simulink model "Team6_1"  (R2018b)
settings: Solver=VariableStepAuto  StartTime=0.0  StopTime=10  RelTol=1e-3
undefined symbols (not defined in the file): sigbuilder_block
(part 1 of 2)
settings Model: EnablePacing=on  PacingRate=0.500000  Creator=99003175  LastModifiedBy=Hp
settings DataIOCC: ReturnWorkspaceOutputs=on
settings OptimizationCC: DefaultUnderspecifiedDataType=single
settings DebuggingCC: SignalInfNanChecking=warning  UniqueDataStoreMsg=error  AssertControl=DisableAll  StrictBusMsg=ErrorOnBusTreatedAsVector  SFUndirectedBroadcastEventsDiag=error
settings SFSimCC: CompileTimeRecursionLimit=0  EnableRuntimeRecursion=off  MATLABDynamicMemAlloc=off

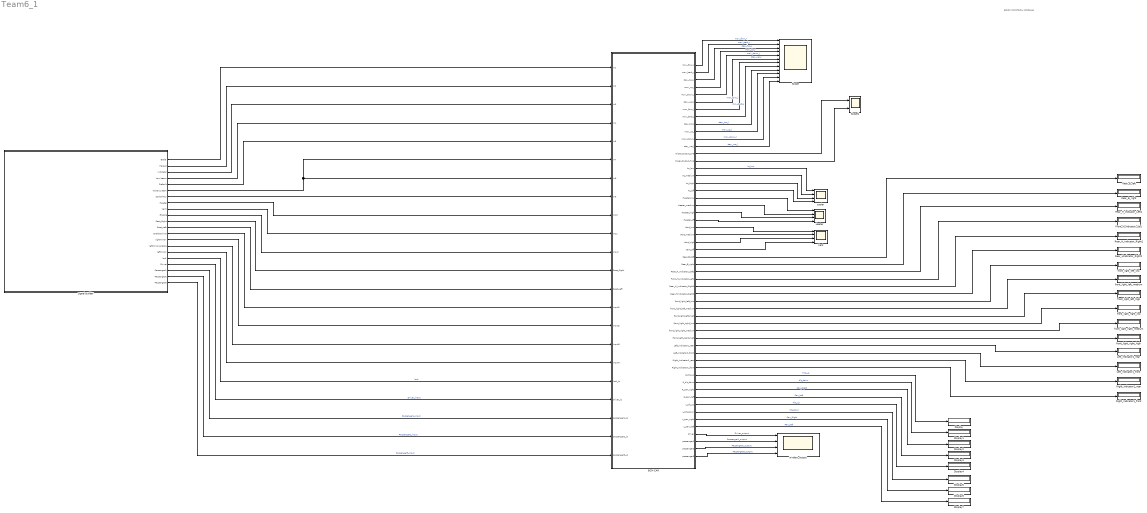
== system Team6_1 ==
  note: BODY CONTROL MODULE
  BCM CAR : Subsystem
  Display{,1..7} (8 alike) : Display
  Front_H_Indicator_Lef1 : Display
  Heater : Scope  NumInputPorts=4
  Left_Indicator1_front : Display
  Left_Indicator1_rear : Display
  Rear_B_left : Display
  Rear_B_right : Display
  Rear_HIndicator_Right2 : Display
  Rear_H_Indicator_Left1 : Display
  Rear_H_Indicator_Right1 : Display
  Right_Indicator1_front : Display
  Right_Indicator1_rear : Display
  Scope : Scope  NumInputPorts=12
  Scope1 : Scope  NumInputPorts=2
  Signal Builder : Subsystem  Tag=STV Subsys  LoadFcn=sigbuilder_block('load');  StartFcn=sigbuilder_block('start');  StopFcn=sigbuilder_block('stop');  ClipboardFcn=sigbuilder_block('clipboard');  mask(Sigbuilder block){tuvar=[0:10]}
      mask help: Simulink:masks:SigbuilderBlock_MD
      mask init:
      | if ~strcmp(get_param(bdroot(gcbh),'SimulationStatus'),'stopped') tuvar = sigbuilder_block('maskInit'); end
      settings: CopyFcn=sigbuilder_block('copy');  DeleteFcn=sigbuilder_block('delete');  ModelCloseFcn=sigbuilder_block('modelClose');  PreSaveFcn=sigbuilder_block('preSave');  PauseFcn=sigbuilder_block('pause');  ContinueFcn=sigbuilder_block('continue');  NameChangeFcn=sigbuilder_block('namechange');  OpenFcn=sigbuilder_block('open',[6 46.5 1188 465.75 ]);  CloseFcn=sigbuilder_block('close');
      mask Display: plot(0, 0, 100, 100,[2, 2, 32, 32, 2], [68, 8, 8, 68, 68],[32, 2], [38, 38], [32, 19, 2],[53, 60, 44], [32, 17, 17, 2],[16, 16, 31, 31]);txt = getActiveGroup(gcbh);text(2, 100, txt,'verticalAlignment', 'top');
  Vent : Scope  NumInputPorts=4
  cooler : Scope  NumInputPorts=4
  front_light_left_high : Display
  front_light_left_low : Display
  front_light_left_medium : Display
  front_light_right_high : Display
  front_light_right_low : Display
  front_light_right_medium : Display
  window_output : Scope  NumInputPorts=4
  wires:
  Signal Builder/9(Vent) -> BCM CAR/10(In11)
  Signal Builder/16(leftmirror) -> BCM CAR/17(Input4)
  BCM CAR/46(R_pan_left) -> Display3/1  "Pan_left"
  Signal Builder/15(leftmirror enable) -> BCM CAR/16(Input3)
  Signal Builder/14(rightmirror) -> BCM CAR/15(Input2)
  BCM CAR/43(R_tilt_up) -> Display/1  "Tilt_up"
  BCM CAR/45(R_pan_right) -> Display2/1  "Pan_Right"
  Signal Builder/13(enablemirror) -> BCM CAR/14(Input1)
  BCM CAR/44(R_tilt_down) -> Display1/1  "tilt_down"
  Signal Builder/6(Wiper system) -> BCM CAR/6(In7), BCM CAR/7(In8)
  Signal Builder/5(Default) -> BCM CAR/5(In5)
  Signal Builder/12(Seat_Left) -> BCM CAR/13(Seat_Left)
  Signal Builder/4(Low beam) -> BCM CAR/4(In4)
  Signal Builder/1(Brake) -> BCM CAR/1(In1)
  Signal Builder/7(Cooler(AC)) -> BCM CAR/8(In9)
  Signal Builder/3(Indicator) -> BCM CAR/3(In3)
  Signal Builder/10(Enable) -> BCM CAR/11(Input)
  Signal Builder/11(Seat_Right) -> BCM CAR/12(Seat_Right)
  Signal Builder/2(Hazard) -> BCM CAR/2(In2)
  Signal Builder/8(Heater) -> BCM CAR/9(In10)
  BCM CAR/27(Rear_B_left) -> Rear_B_left/1
  BCM CAR/26(Vent_off) -> Vent/4
  BCM CAR/32(Rear_HIndicator_Right2) -> Rear_HIndicator_Right2/1
  BCM CAR/9(stay_hor_l) -> Scope/9  "stay_hor_l"
  BCM CAR/33(front_light_left_low) -> front_light_left_low/1
  BCM CAR/39(Left_Indicator1_rear) -> Left_Indicator1_rear/1
  BCM CAR/30(Front_H_Indicator_Lef1) -> Front_H_Indicator_Lef1/1
  BCM CAR/17(Ac_high) -> cooler/3
  BCM CAR/36(front_light_right_low) -> front_light_right_low/1
  BCM CAR/42(Right_Indicator1_front) -> Right_Indicator1_front/1
  BCM CAR/35(front_light_left_high) -> front_light_left_high/1
  BCM CAR/38(front_light_right_high) -> front_light_right_high/1
  BCM CAR/28(Rear_B_right) -> Rear_B_right/1
  BCM CAR/13(Wiper_Output_one) -> Scope1/1
  BCM CAR/29(Rear_H_Indicator_Left1) -> Rear_H_Indicator_Left1/1
  BCM CAR/31(Rear_H_Indicator_Right1) -> Rear_H_Indicator_Right1/1
  BCM CAR/2(mov_back_r) -> Scope/2  "mov_back_r"
  BCM CAR/3(stay_hor_r) -> Scope/3  "stay_hor_r"
  BCM CAR/37(front_light_right_medium) -> front_light_right_medium/1
  BCM CAR/8(mov_back_l) -> Scope/8  "mov_back_l"
  BCM CAR/34(front_light_left_medium) -> front_light_left_medium/1
  BCM CAR/14(Wiper_Output_Two) -> Scope1/2
  BCM CAR/18(Ac_off) -> cooler/4
  BCM CAR/41(Right_Indicator1_rear) -> Right_Indicator1_rear/1
  BCM CAR/40(Left_Indicator1_front) -> Left_Indicator1_front/1
  BCM CAR/25(Vent_high) -> Vent/3
  BCM CAR/24(Vent_medium) -> Vent/2
  BCM CAR/15(Ac_low) -> cooler/1  "Ac_low"
  BCM CAR/23(Vent_low) -> Vent/1
  BCM CAR/1(mov_forw_r) -> Scope/1  "mov_forw_r"
  BCM CAR/22(Heater_off) -> Heater/4
  BCM CAR/12(stay_ver_l) -> Scope/12  "stay_ver_l"
  BCM CAR/21(Heater_high) -> Heater/3
  BCM CAR/11(mov_down_l) -> Scope/11  "mov_down_l"
  BCM CAR/20(Heater_medium) -> Heater/2
  BCM CAR/19(Heater_low) -> Heater/1
  BCM CAR/16(Ac_medium) -> cooler/2
  BCM CAR/5(mov_down_r) -> Scope/5  "mov_down_r"
  BCM CAR/4(mov_up_r) -> Scope/4  "mov_up_r"
  BCM CAR/6(stay_ver_r) -> Scope/6  "stay_ver_r"
  BCM CAR/7(mov_forw_l) -> Scope/7  "mov_forw_l"
  BCM CAR/10(mov_up_l) -> Scope/10  "mov_up_l"
  BCM CAR/47(L_tilt_up) -> Display4/1  "Tilt_up"
  BCM CAR/50(L_pan_left) -> Display7/1  "Pan_left"
  BCM CAR/49(L_pan_right) -> Display6/1  "Pan_Right"
  BCM CAR/48(L_tilt_down) -> Display5/1  "tilt_down"
  Signal Builder/17(lock) -> BCM CAR/18(lock_ip)  "lock"
  Signal Builder/18(Driver) -> BCM CAR/19(driver_ip)  "Driver_input"
  Signal Builder/19(Passenger1) -> BCM CAR/20(passenger1_ip)  "Passenger1_input"
  Signal Builder/20(Passenger2) -> BCM CAR/21(passenger2_ip)  "Passenger2_input"
  Signal Builder/21(Passenger3) -> BCM CAR/22(passenger3_ip)  "Passenger3_input"
  BCM CAR/51(driver) -> window_output/1  "Driver_output"
  BCM CAR/52(passenger1) -> window_output/2  "Passenger1_output"
  BCM CAR/53(passenger2) -> window_output/3  "Passenger2_output"
  BCM CAR/54(passenger3) -> window_output/4  "Passenger3_output"

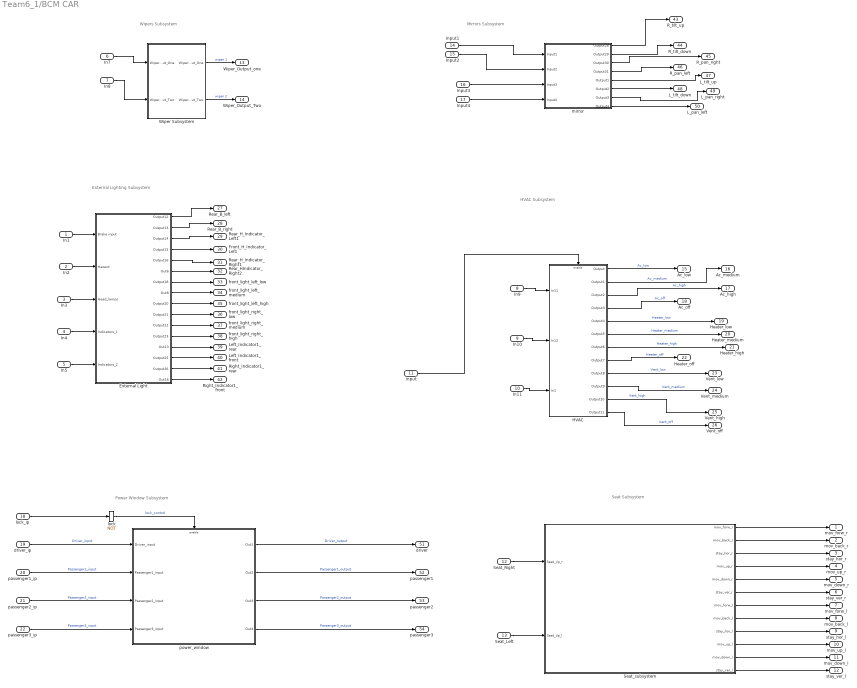
== system Team6_1/BCM CAR ==
  note: Seat Subsystem
  note: External Lighting Subsystem
  note: HVAC Subsystem
  note: Mirrors Subsystem
  note: Wipers Subsystem
  note: Power Window Subsystem
  In1 : Inport
  In2 : Inport  Port=2
  In3 : Inport  Port=3
  In4 : Inport  Port=4
  In5 : Inport  Port=5
  In7 : Inport  Port=6
  In8 : Inport  Port=7
  In9 : Inport  Port=8
  In10 : Inport  Port=9
  In11 : Inport  Port=10
  Input : Inport  Port=11
  Seat_Right : Inport  Port=12
  Seat_Left : Inport  Port=13
  Input1 : Inport  Port=14
  Input2 : Inport  Port=15
  Input3 : Inport  Port=16
  Input4 : Inport  Port=17
  lock_ip : Inport  Port=18
  driver_ip : Inport  Port=19
  passenger1_ip : Inport  Port=20
  passenger2_ip : Inport  Port=21
  passenger3_ip : Inport  Port=22
  External Light : Subsystem  TreatAsAtomicUnit=on
  HVAC : Subsystem
  Seat_subsystem : Subsystem  TreatAsAtomicUnit=on
  Wiper Subsystem : Subsystem  TreatAsAtomicUnit=on
  lock : Logic  Operator=NOT  IconShape=distinctive  AllPortsSameDT=off  OutDataTypeStr=boolean
  mirror : Subsystem  TreatAsAtomicUnit=on
  power_window : Subsystem
  mov_forw_r : Outport
  mov_back_r : Outport  Port=2
  stay_hor_r : Outport  Port=3
  mov_up_r : Outport  Port=4
  mov_down_r : Outport  Port=5
  stay_ver_r : Outport  Port=6
  mov_forw_l : Outport  Port=7
  mov_back_l : Outport  Port=8
  stay_hor_l : Outport  Port=9
  mov_up_l : Outport  Port=10
  mov_down_l : Outport  Port=11
  stay_ver_l : Outport  Port=12
  Wiper_Output_one : Outport  Port=13
  Wiper_Output_Two : Outport  Port=14
  Ac_low : Outport  Port=15
  Ac_medium : Outport  Port=16
  Ac_high : Outport  Port=17
  Ac_off : Outport  Port=18
  Heater_low : Outport  Port=19
  Heater_medium : Outport  Port=20
  Heater_high : Outport  Port=21
  Heater_off : Outport  Port=22
  Vent_low : Outport  Port=23
  Vent_medium : Outport  Port=24
  Vent_high : Outport  Port=25
  Vent_off : Outport  Port=26
  Rear_B_left : Outport  Port=27
  Rear_B_right : Outport  Port=28
  Rear_H_Indicator_Left1 : Outport  Port=29
  Front_H_Indicator_Lef1 : Outport  Port=30
  Rear_H_Indicator_Right1 : Outport  Port=31
  Rear_HIndicator_Right2 : Outport  Port=32
  front_light_left_low : Outport  Port=33
  front_light_left_medium : Outport  Port=34
  front_light_left_high : Outport  Port=35
  front_light_right_low : Outport  Port=36
  front_light_right_medium : Outport  Port=37
  front_light_right_high : Outport  Port=38
  Left_Indicator1_rear : Outport  Port=39
  Left_Indicator1_front : Outport  Port=40
  Right_Indicator1_rear : Outport  Port=41
  Right_Indicator1_front : Outport  Port=42
  R_tilt_up : Outport  Port=43
  R_tilt_down : Outport  Port=44
  R_pan_right : Outport  Port=45
  R_pan_left : Outport  Port=46
  L_tilt_up : Outport  Port=47
  L_tilt_down : Outport  Port=48
  L_pan_right : Outport  Port=49
  L_pan_left : Outport  Port=50
  driver : Outport  Port=51
  passenger1 : Outport  Port=52
  passenger2 : Outport  Port=53
  passenger3 : Outport  Port=54
  wires:
  In7/1 -> Wiper Subsystem/1(Wiper_Input_One)
  HVAC/6(Output5) -> Heater_medium/1  "Heater_medium"
  HVAC/3(Output2) -> Ac_high/1  "Ac_high"
  In1/1 -> External Light/1(Brake input)
  HVAC/7(Output6) -> Heater_high/1  "Heater_high"
  In4/1 -> External Light/4(Indicators_1)
  HVAC/4(Output3) -> Ac_off/1  "Ac_off"
  In8/1 -> Wiper Subsystem/2(Wiper_Input_Two)
  In9/1 -> HVAC/1(In11)
  HVAC/2(Output1) -> Ac_medium/1  "Ac_medium"
  HVAC/5(Output4) -> Heater_low/1  "Heater_low"
  In10/1 -> HVAC/2(In12)
  HVAC/12(Output11) -> Vent_off/1  "Vent_off"
  HVAC/10(Output9) -> Vent_medium/1  "Vent_medium"
  In5/1 -> External Light/5(Indicators_2)
  HVAC/8(Output7) -> Heater_off/1  "Heater_off"
  HVAC/11(Output10) -> Vent_high/1  "Vent_high"
  HVAC/1(Output) -> Ac_low/1  "Ac_low"
  HVAC/9(Output8) -> Vent_low/1  "Vent_low"
  In11/1 -> HVAC/3(In1)
  In3/1 -> External Light/3(Head_lamps)
  In2/1 -> External Light/2(Hazard)
  Input/1 -> HVAC/Enable
  Seat_subsystem/7(mov_forw_l) -> mov_forw_l/1
  Seat_subsystem/8(mov_back_l) -> mov_back_l/1
  Seat_subsystem/6(stay_ver_r) -> stay_ver_r/1
  Seat_Right/1 -> Seat_subsystem/1(Seat_i/p_r)
  Seat_Left/1 -> Seat_subsystem/2(Seat_i/p_l)
  Seat_subsystem/9(stay_hor_l) -> stay_hor_l/1
  Seat_subsystem/11(mov_down_l) -> mov_down_l/1
  Seat_subsystem/12(stay_ver_l) -> stay_ver_l/1
  Seat_subsystem/4(mov_up_r) -> mov_up_r/1
  Seat_subsystem/1(mov_forw_r) -> mov_forw_r/1
  Seat_subsystem/5(mov_down_r) -> mov_down_r/1
  Seat_subsystem/3(stay_hor_r) -> stay_hor_r/1
  Seat_subsystem/10(mov_up_l) -> mov_up_l/1
  Seat_subsystem/2(mov_back_r) -> mov_back_r/1
  Wiper Subsystem/1(Wiper_Output_One) -> Wiper_Output_one/1  "wiper 1"
  Wiper Subsystem/2(Wiper_Output_Two) -> Wiper_Output_Two/1  "wiper 2"
  External Light/1(Output12) -> Rear_B_left/1
  External Light/2(Output13) -> Rear_B_right/1
  External Light/3(Output14) -> Rear_H_Indicator_Left1/1
  External Light/4(Output15) -> Front_H_Indicator_Lef1/1
  External Light/5(Output16) -> Rear_H_Indicator_Right1/1
  External Light/6(Out6) -> Rear_HIndicator_Right2/1
  External Light/7(Output18) -> front_light_left_low/1
  External Light/8(Out8) -> front_light_left_medium/1
  External Light/9(Output20) -> front_light_left_high/1
  External Light/10(Output21) -> front_light_right_low/1
  External Light/11(Output22) -> front_light_right_medium/1
  External Light/12(Output23) -> front_light_right_high/1
  External Light/13(Out13) -> Left_Indicator1_rear/1
  External Light/14(Output25) -> Left_Indicator1_front/1
  External Light/15(Output26) -> Right_Indicator1_rear/1
  External Light/16(Out16) -> Right_Indicator1_front/1
  Input1/1 -> mirror/1(Input1)
  Input2/1 -> mirror/2(Input2)
  mirror/1(Output28) -> R_tilt_up/1
  mirror/3(Output30) -> R_pan_right/1
  mirror/2(Output29) -> R_tilt_down/1
  mirror/4(Output31) -> R_pan_left/1
  mirror/5(Output1) -> L_tilt_up/1
  mirror/6(Output2) -> L_tilt_down/1
  mirror/7(Output3) -> L_pan_right/1
  mirror/8(Output4) -> L_pan_left/1
  Input4/1 -> mirror/4(Input4)
  Input3/1 -> mirror/3(Input3)
  lock/1 -> power_window/Enable  "lock_control"
  passenger1_ip/1 -> power_window/2(Passenger1_input)  "Passenger1_input"
  power_window/3(Out3) -> passenger2/1  "Passenger2_output"
  power_window/2(Out2) -> passenger1/1  "Passenger1_output"
  passenger3_ip/1 -> power_window/4(Passenger3_input)  "Passenger3_input"
  passenger2_ip/1 -> power_window/3(Passenger2_input)  "Passenger2_input"
  driver_ip/1 -> power_window/1(Driver_input)  "Driver_input"
  power_window/1(Out1) -> driver/1  "Driver_output"
  power_window/4(Out4) -> passenger3/1  "Passenger3_output"
  lock_ip/1 -> lock/1

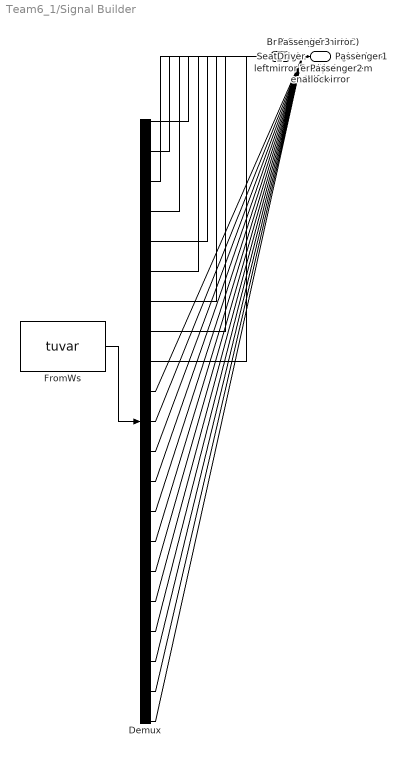
== system Team6_1/Signal Builder ==
  Demux : Demux  Tag=STV Demux  Outputs=21
      settings: DisplayOption=none
  FromWs : FromWorkspace  Tag=STV FromWs  VariableName=tuvar
      SigBuilderData=|
      | common.afterFinalStr = 'Extrapolate'
      | common.sampleTime = 0
      | dataSet.timeRange = [0 10]
      | dataSet.name = 'Group 1'
      | sbobj.Groups.Name = 'Group 1'
      | sbobj.Groups.Signals(1).Name = 'Brake'
      | sbobj.Groups.Signals(1).XData = [0 3 3 6 6 10]
      | sbobj.Groups.Signals(1).YData = [0 0 1 1 0 0]
      | sbobj.Groups.Signals(2).Name = 'Hazard'
      | sbobj.Groups.Signals(2).XData = [0 0.5 0.5 1 1 1.5 1.5 2 2 2.5 2.5 3 3 3.5 3.5 4 4 4.5 4.5 5 5 5.5 5.5 6 6 6.5 6.5 7 7 7.5 7.5 8 8 8.5 8.5 9 9 9.5 9.5 10]
      | sbobj.Groups.Signals(2).YData = [2 2 0 0 2 2 0 0 2 2 0 0 2 2 0 0 2 2 0 0 2 2 0 0 2 2 0 0 2 2 0 0 2 2 0 0 2 2 0 0]
      | sbobj.Groups.Signals(3).Name = 'Indicator'
      | sbobj.Groups.Signals(3).XData = [0 1 1 4.02 4.02 10]
      | sbobj.Groups.Signals(3).YData = [0 0 1.05 1.05 0 0]
      | sbobj.Groups.Signals(4).Name = 'Low beam'
      | sbobj.Groups.Signals(4).XData = [0 5.96 5.96 7.96 7.96 10]
      | sbobj.Groups.Signals(4).YData = [0 0 1.05 1.05 0 0]
      | sbobj.Groups.Signals(5).Name = 'Default'
      | sbobj.Groups.Signals(5).XData = [0 1 1 8 8 10]
      | sbobj.Groups.Signals(5).YData = [0 0 -0.4 -0.4 1 1]
      | sbobj.Groups.Signals(6).Name = 'Wiper system'
      | sbobj.Groups.Signals(6).XData = [0 0.5 1 1 1.5 1.5 2 2 2.5 2.5 3 3 3.5 3.5 4 4 4.5 4.5 5 5 5.5 5.5 6 6 6.5 6.5 7 7 7.5 7.5 8 8 8.5 8.5 9 9 9.5 9.5 10]
      | sbobj.Groups.Signals(6).YData = [3 3 3 2.5 1 2 2 0.85 0.85 1.95 1.95 1 1 1.1 1.1 2 2 0.95 0.95 0.8 0.8 0.95 0.95 2 2 0.8 0.8 2.5 2.5 2.05 2.05 0.95 0.95 0.6 0.6 0 0 5 5]
      | sbobj.Groups.Signals(7).Name = 'Cooler(AC)'
      | sbobj.Groups.Signals(7).XData = [0 0.5 0.5 1 1 1.5 1.5 2 2 2.5 2.5 3 3 3.5 3.5 4 4 4.5 4.5 5 5 5.5 5.5 6 6 6.5 6.5 7 7 7.5 7.5 8 8 8.5 8.5 9 9 9.5 10]
      | sbobj.Groups.Signals(7).YData = [2 2 1 1 0 0 0.9 0.9 2 2 3 3 1.2 1.2 2.2 2.2 0.9 0.9 0 0 2 2 3 3 2 2 0 0 2 2 0 0 2 2 0 0 2 2 2]
      | sbobj.Groups.Signals(8).Name = 'Heater'
      | sbobj.Groups.Signals(8).XData = [0 0.5 0.5 1 1 1.5 1.5 2 2 2.5 2.5 3 3 3.5 3.5 4 4 4.5 4.5 5 5 5.5 5.5 6 6 6.5 6.5 7 7 7.5 7.5 8 8 8.5 8.5 9 9 9.5 9.5 10]
      | sbobj.Groups.Signals(8).YData = [2 2 0.9 0.9 0 0 0.8 0.8 2 2 0 0 3 3 1 1 2 2 0 0 1 1 0 0 3 3 2 2 3 3 0 0 2 2 0 0 2 2 1 1]
      | sbobj.Groups.Signals(9).Name = 'Vent'
      | sbobj.Groups.Signals(9).XData = [0 0.5 0.5 1 1 1.5 1.5 2 2 2.5 2.5 3 3 3.5 3.5 4 4 4.5 4.5 5 5 5.5 5.5 6 6 6.5 6.5 7 7 7.5 7.5 8 8 8.5 8.5 9 9 9.5 9.5 10]
      | sbobj.Groups.Signals(9).YData = [2 2 1.1 1.1 0 0 1.8 1.8 0.9 0.9 1.9 1.9 0.1 0.1 1.8 1.8 -0.2 -0.2 1.4 1.4 3 3 0 0 2 2 3 3 2 2 1 1 2 2 0 0 3 3 1.1 1.1]
      | sbobj.Groups.Signals(10).Name = 'Enable'
      | sbobj.Groups.Signals(10).XData = [0 10]
      | sbobj.Groups.Signals(10).YData = [1 1]
      | sbobj.Groups.Signals(11).Name = 'Seat_Right'
      | sbobj.Groups.Signals(11).XData = [0 0.5 0.5 1 1 1.5 1.5 2 2 2.5 2.5 3 3 3.5 3.5 4 4 4.5 4.5 5 5 5.5 5.5 6 6 6.5 6.5 7 7 7.5 7.5 8 8 8.5 8.5 9 9 9.5 9.5 10]
      | sbobj.Groups.Signals(11).YData = [1 1 0 0 1 1 -1 -1 1 1 0 0 1 1 0 0 1 1 0 0 2 2 0 0 2 2 0 0 2 2 0 0 2 2 0 0 2 2 0 0]
      | sbobj.Groups.Signals(12).Name = 'Seat_Left'
      | sbobj.Groups.Signals(12).XData = [0 0.5 0.5 1 1 1.5 1.5 2 2 2.5 2.5 3 3 3.5 3.5 4 4 4.5 4.5 5 5 5.5 5.5 6 6 6.5 6.5 7 7 7.5 7.5 8 8 8.5 8.5 9 9 9.5 9.5 10]
      | sbobj.Groups.Signals(12).YData = [1 1 0 0 -1 -1 0 0 1 1 0 0 -1 -1 0 0 1 1 0 0 2 2 0 0 2 2 0 0 2 2 0 0 2 2 0 0 2 2 0 0]
      | sbobj.Groups.Signals(13).Name = 'enablemirror'
      | sbobj.Groups.Signals(13).XData = [0 0.5 0.5 1 1 1.5 1.5 2 2.5 3 3 3.5 3.5 4 4 4.5 4.5 5 5 5.5 5.5 6 6 6.5 6.5 7 7 7.5 7.5 8 8 8.5 8.5 9 9 9.5 9.5 10]
      | sbobj.Groups.Signals(13).YData = [1 1 0 0 -1 -1 0 0 0 0 1 1 0 0 -1 -1 0 0 2 2 0 0 2 2 0 0 2 2 0 0 2 2 0 0 2 2 0 0]
      | sbobj.Groups.Signals(14).Name = 'rightmirror'
      | sbobj.Groups.Signals(14).XData = [0 0.5 0.5 1 1 1.5 1.5 2 2 2.5 2.5 3 3 3.5 3.5 4 4 4.5 4.5 5 5 5.5 5.5 6 6 6.5 6.5 7 7 7.5 7.5 8 8 8.5 8.5 9 9 9.5 9.5 10]
      | sbobj.Groups.Signals(14).YData = [2 2 0 0 -1 -1 1 1 2 2 0 0 1 1 -1 -1 2 2 0 0 1 1 -1 -1 2 2 1 1 2 2 0 0 1 1 0 0 -1 -1 1 1]
      | sbobj.Groups.Signals(15).Name = 'leftmirror enable'
      | sbobj.Groups.Signals(15).XData = [0 10]
      | sbobj.Groups.Signals(15).YData = [1 1]
      | sbobj.Groups.Signals(16).Name = 'leftmirror'
      | sbobj.Groups.Signals(16).XData = [0 0.5 0.5 1 1 1.5 1.5 2 2 2.5 2.5 3 3 3.5 3.5 4 4 4.5 4.5 5 5 5.5 5.5 6 6 6.5 6.5 7 7 7.5 7.5 8 8 8.5 8.5 9 9 9.5 9.5 10]
      | sbobj.Groups.Signals(16).YData = [2 2 0 0 2 2 0 0 2 2 0 0 2 2 0 0 2 2 0 0 2 2 0 0 2 2 0 0 2 2 0 0 2 2 0 0 2 2 0 0]
      | sbobj.Groups.Signals(17).Name = 'lock'
      | sbobj.Groups.Signals(17).XData = [0 0.5 1 1 1.5 1.5 2 2 2.5 2.5 3 3 3.5 3.5 4 4 4.5 4.5 5 5 5.5 5.5 6 6 6.5 6.5 7 7 7.5 7.5 8 8 8.5 8.5 9 9 9.5 9.5 10]
      | sbobj.Groups.Signals(17).YData = [0 0 0 1 1 0 0 1 1 0 0 2 2 0 0 2 2 0 0 2 2 0 0 2 2 0 0 2 2 0 0 2 2 0 0 2 2 0 0]
      | sbobj.Groups.Signals(18).Name = 'Driver'
      | sbobj.Groups.Signals(18).XData = [0 0.5 1 1 1.5 1.5 2 2 2.5 2.5 3 3 3.5 3.5 4 4 4.5 4.5 5 5 5.5 5.5 6 6 6.5 6.5 7 7 7.5 7.5 8 8 8.5 8.5 9 9 9.5 9.5 10]
      | sbobj.Groups.Signals(18).YData = [1 1 1 2 2 0 0 3 3 0 0 4 4 0 0 2 2 0 0 2 2 0 0 2 2 0 0 2 2 0 0 2 2 0 0 2 2 0 0]
      | sbobj.Groups.Signals(19).Name = 'Passenger1'
      | sbobj.Groups.Signals(19).XData = [0 0.5 0.5 1 1 1.5 1.5 2 2 2.5 2.5 3 3 3.5 3.5 4 4 4.5 4.5 5 5 5.5 5.5 6 6 6.5 6.5 7 7 7.5 7.5 8 8 8.5 8.5 9 9 9.5 9.5 10]
      | sbobj.Groups.Signals(19).YData = [1 1 0 0 2 2 0 0 3 3 0 0 4 4 0 0 2 2 0 0 2 2 0 0 2 2 0 0 2 2 0 0 2 2 0 0 2 2 0 0]
      | sbobj.Groups.Signals(20).Name = 'Passenger2'
      | sbobj.Groups.Signals(20).XData = [0 0.5 0.5 1 1 1.5 1.5 2 2 2.5 2.5 3 3 3.5 3.5 4 4 4.5 4.5 5 5 5.5 5.5 6 6 6.5 6.5 7 7 7.5 7.5 8 8 8.5 8.5 9 9 9.5 9.5 10]
      | sbobj.Groups.Signals(20).YData = [1 1 0 0 2 2 0 0 3 3 0 0 4 4 0 0 2 2 0 0 2 2 0 0 2 2 0 0 2 2 0 0 2 2 0 0 2 2 0 0]
      | sbobj.Groups.Signals(21).Name = 'Passenger3'
      | sbobj.Groups.Signals(21).XData = [0 0.5 0.5 1 1 1.5 1.5 2 2 2.5 2.5 3 3 3.5 3.5 4 4 4.5 4.5 5 5 5.5 5.5 6 6 6.5 6.5 7 7 7.5 7.5 8 8 8.5 8.5 9 9 9.5 9.5 10]
      | sbobj.Groups.Signals(21).YData = [1 1 0 0 2 2 0 0 3 3 0 0 4 4 0 0 2 2 0 0 2 2 0 0 2 2 0 0 2 2 0 0 2 2 0 0 2 2 0 0]
  Brake : Outport  Tag=STV Outport
  Hazard : Outport  Tag=STV Outport  Port=2
  Indicator : Outport  Tag=STV Outport  Port=3
  Low beam : Outport  Tag=STV Outport  Port=4
  Default : Outport  Tag=STV Outport  Port=5
  Wiper system : Outport  Tag=STV Outport  Port=6
  Cooler(AC) : Outport  Tag=STV Outport  Port=7
  Heater : Outport  Tag=STV Outport  Port=8
  Vent : Outport  Tag=STV Outport  Port=9
  Enable : Outport  Tag=STV Outport  Port=10
  Seat_Right : Outport  Tag=STV Outport  Port=11
  Seat_Left : Outport  Tag=STV Outport  Port=12
  enablemirror : Outport  Tag=STV Outport  Port=13
  rightmirror : Outport  Tag=STV Outport  Port=14
  leftmirror enable : Outport  Tag=STV Outport  Port=15
  leftmirror : Outport  Tag=STV Outport  Port=16
  lock : Outport  Tag=STV Outport  Port=17
  Driver : Outport  Tag=STV Outport  Port=18
  Passenger1 : Outport  Tag=STV Outport  Port=19
  Passenger2 : Outport  Tag=STV Outport  Port=20
  Passenger3 : Outport  Tag=STV Outport  Port=21
  wires:
  Demux/1 -> Brake/1
  FromWs/1 -> Demux/1
  Demux/2 -> Hazard/1
  Demux/3 -> Indicator/1
  Demux/4 -> Low beam/1
  Demux/5 -> Default/1
  Demux/6 -> Wiper system/1
  Demux/7 -> Cooler(AC)/1
  Demux/8 -> Heater/1
  Demux/9 -> Vent/1
  Demux/10 -> Enable/1
  Demux/11 -> Seat_Right/1
  Demux/12 -> Seat_Left/1
  Demux/13 -> enablemirror/1
  Demux/14 -> rightmirror/1
  Demux/15 -> leftmirror enable/1
  Demux/16 -> leftmirror/1
  Demux/17 -> lock/1
  Demux/18 -> Driver/1
  Demux/19 -> Passenger1/1
  Demux/20 -> Passenger2/1
  Demux/21 -> Passenger3/1

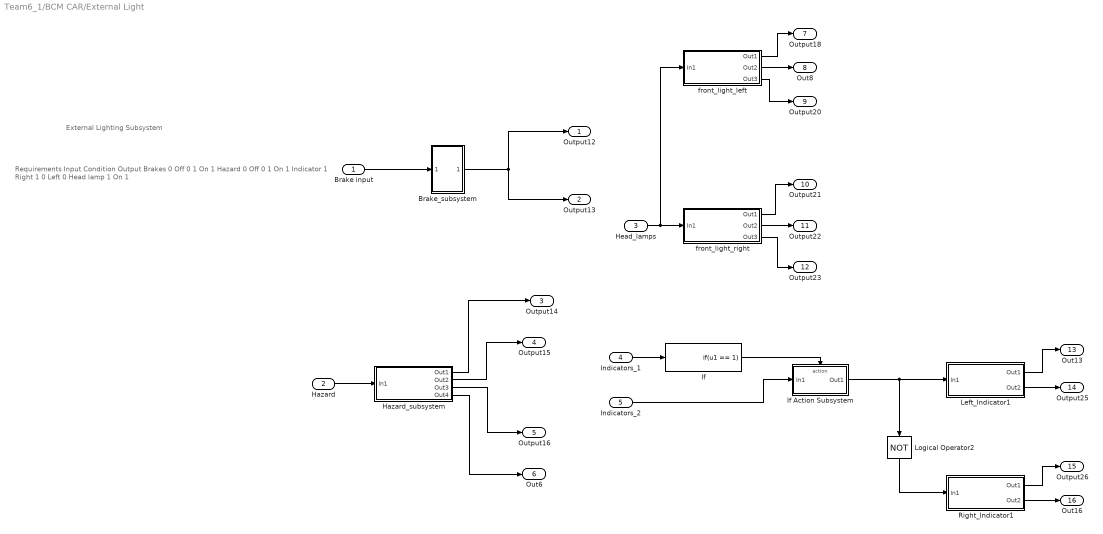
== system Team6_1/BCM CAR/External Light ==
  note: Requirements
      | Input
      | Condition
      | Output
      |
      | Brakes
      | 0
      | Off
      | 0
      |
      | 1
      | On
      | 1
      |
      | Hazard
      | 0
      | Off
      | 0
      |
      | 1
      | On
      | 1
      |
      | Indicator
      | 1
      | Right
      | 1
      |
      | 0
      | Left
      | 0
      |
      | Head lamp
      | 1
      | On
      | 1
  note: External Lighting Subsystem
  Brake input : Inport
  Hazard : Inport  Port=2
  Head_lamps : Inport  Port=3
  Indicators_1 : Inport  Port=4
  Indicators_2 : Inport  Port=5
  Brake_subsystem : Subsystem
  Hazard_subsystem : Subsystem
  If : If  IfExpression=u1 == 1  ShowElse=off
  If Action Subsystem : Subsystem  TreatAsAtomicUnit=on
  Left_Indicator1 : Subsystem
  Logical Operator2 : Logic  Operator=NOT  AllPortsSameDT=off  OutDataTypeStr=boolean
  Right_Indicator1 : Subsystem
  front_light_left : Subsystem
  front_light_right : Subsystem
  Output12 : Outport
  Output13 : Outport  Port=2
  Output14 : Outport  Port=3
  Output15 : Outport  Port=4
  Output16 : Outport  Port=5
  Out6 : Outport  Port=6
  Output18 : Outport  Port=7
  Out8 : Outport  Port=8
  Output20 : Outport  Port=9
  Output21 : Outport  Port=10
  Output22 : Outport  Port=11
  Output23 : Outport  Port=12
  Out13 : Outport  Port=13
  Output25 : Outport  Port=14
  Output26 : Outport  Port=15
  Out16 : Outport  Port=16
  wires:
  Hazard_subsystem/1(Out1) -> Output14/1
  Hazard_subsystem/4(Out4) -> Out6/1
  Hazard_subsystem/2(Out2) -> Output15/1
  Hazard_subsystem/3(Out3) -> Output16/1
  Hazard/1 -> Hazard_subsystem/1(In1)
  Brake_subsystem/1(Out1) -> Output13/1, Output12/1
  Brake input/1 -> Brake_subsystem/1(In1)
  front_light_left/1(Out1) -> Output18/1
  If/1 -> If Action Subsystem/Action
  front_light_left/3(Out3) -> Output20/1
  front_light_left/2(Out2) -> Out8/1
  If Action Subsystem/1(Out1) -> Logical Operator2/1, Left_Indicator1/1(In1)
  Left_Indicator1/2(Out2) -> Output25/1
  Logical Operator2/1 -> Right_Indicator1/1(In1)
  Head_lamps/1 -> front_light_left/1(In1), front_light_right/1(In1)
  Right_Indicator1/2(Out2) -> Out16/1
  Right_Indicator1/1(Out1) -> Output26/1
  Indicators_1/1 -> If/1
  front_light_right/2(Out2) -> Output22/1
  front_light_right/1(Out1) -> Output21/1
  Indicators_2/1 -> If Action Subsystem/1(In1)
  Left_Indicator1/1(Out1) -> Out13/1
  front_light_right/3(Out3) -> Output23/1

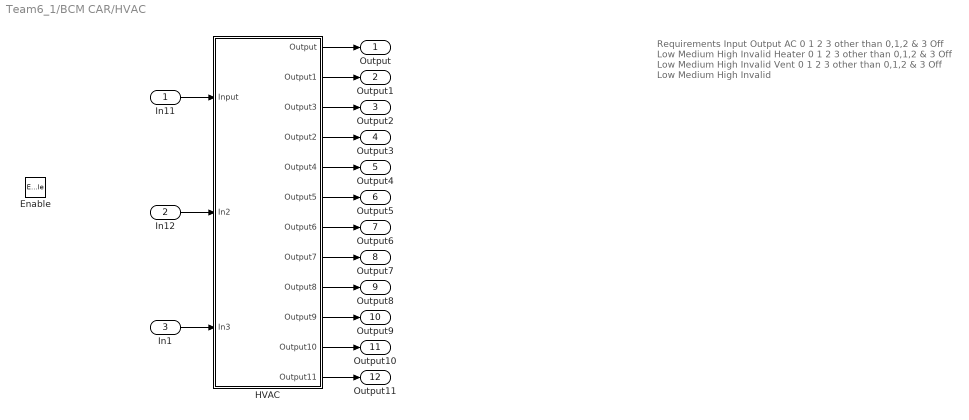
== system Team6_1/BCM CAR/HVAC ==
  note: Requirements
      | Input
      | Output
      |
      | AC
      | 0
      | 1
      | 2
      | 3
      | other than 0,1,2 & 3
      | Off
      | Low
      | Medium
      | High
      | Invalid
      |
      | Heater
      | 0
      | 1
      | 2
      | 3
      | other than 0,1,2 & 3
      | Off
      | Low
      | Medium
      | High
      | Invalid
      |
      | Vent
      | 0
      | 1
      | 2
      | 3
      | other than 0,1,2 & 3
      | Off
      | Low
      | Medium
      | High
      | Invalid
  In11 : Inport
  In12 : Inport  Port=2
  In1 : Inport  Port=3
  Enable : EnablePort
  HVAC : Subsystem
  Output : Outport
  Output1 : Outport  Port=2
  Output2 : Outport  Port=3
  Output3 : Outport  Port=4
  Output4 : Outport  Port=5
  Output5 : Outport  Port=6
  Output6 : Outport  Port=7
  Output7 : Outport  Port=8
  Output8 : Outport  Port=9
  Output9 : Outport  Port=10
  Output10 : Outport  Port=11
  Output11 : Outport  Port=12
  wires:
  HVAC/11(Output10) -> Output10/1
  HVAC/4(Output2) -> Output3/1
  HVAC/3(Output3) -> Output2/1
  HVAC/5(Output4) -> Output4/1
  HVAC/6(Output5) -> Output5/1
  In11/1 -> HVAC/1(Input)
  HVAC/7(Output6) -> Output6/1
  HVAC/2(Output1) -> Output1/1
  HVAC/8(Output7) -> Output7/1
  HVAC/1(Output) -> Output/1
  HVAC/9(Output8) -> Output8/1
  In1/1 -> HVAC/3(In3)
  HVAC/10(Output9) -> Output9/1
  In12/1 -> HVAC/2(In2)
  HVAC/12(Output11) -> Output11/1

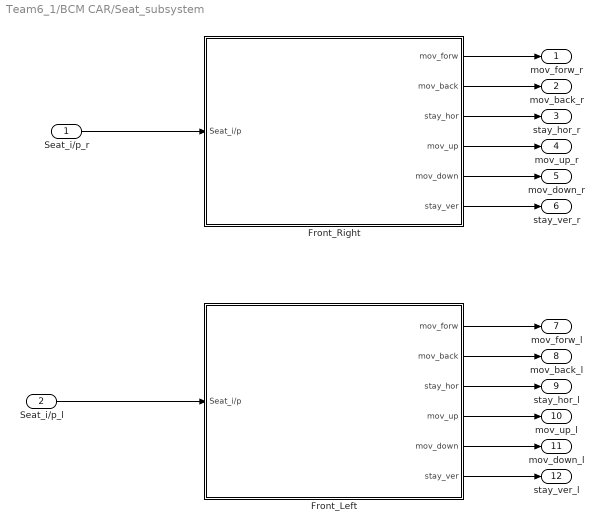
== system Team6_1/BCM CAR/Seat_subsystem ==
  Seat_i/p_r : Inport
  Seat_i/p_l : Inport  Port=2
  Front_Left : Subsystem  TreatAsAtomicUnit=on
  Front_Right : Subsystem  TreatAsAtomicUnit=on
  mov_forw_r : Outport
  mov_back_r : Outport  Port=2
  stay_hor_r : Outport  Port=3
  mov_up_r : Outport  Port=4
  mov_down_r : Outport  Port=5
  stay_ver_r : Outport  Port=6
  mov_forw_l : Outport  Port=7
  mov_back_l : Outport  Port=8
  stay_hor_l : Outport  Port=9
  mov_up_l : Outport  Port=10
  mov_down_l : Outport  Port=11
  stay_ver_l : Outport  Port=12
  wires:
  Seat_i/p_r/1 -> Front_Right/1(Seat_i/p)
  Front_Right/2(mov_back) -> mov_back_r/1
  Front_Right/1(mov_forw) -> mov_forw_r/1
  Front_Right/3(stay_hor) -> stay_hor_r/1
  Front_Right/4(mov_up) -> mov_up_r/1
  Front_Right/5(mov_down) -> mov_down_r/1
  Front_Right/6(stay_ver) -> stay_ver_r/1
  Front_Left/1(mov_forw) -> mov_forw_l/1
  Front_Left/2(mov_back) -> mov_back_l/1
  Front_Left/3(stay_hor) -> stay_hor_l/1
  Front_Left/4(mov_up) -> mov_up_l/1
  Front_Left/5(mov_down) -> mov_down_l/1
  Front_Left/6(stay_ver) -> stay_ver_l/1
  Seat_i/p_l/1 -> Front_Left/1(Seat_i/p)

== system Team6_1/BCM CAR/Wiper Subsystem ==
  note: Requirements
      | 1- There are two subsytems. As
      | there are two wipers in a car.
      | 2- The input is same for both
      | the subsystems.
      | 3- The input of the system is as fallows
      | 0 for off
      | 1 for low speed
      | 2 for medium speed
      | 3 for high speed
      | 2- The output is given to scope. The output is
      | varies is 0,20,40 and 60
  note: Test Plan
  note: Sl No.
      | Test Cases
      | Input
      | output
      | Result
      |
      | 1.
      | Slow Speed
      | 1
      | A Signal of frequency 1
      | PASS
      |
      | 2.
      | Medium Speed
      | 2
      | A signal of frequency
      | 2
      | PASS
      |
      | 3.
      | High speed
      | 3
      | A Signal of frequency
      | 3
      | PASS
      |
      | 4.
      | OFF
      | 0
      | 0
      | PASS
  Wiper_Input_One : Inport
  Wiper_Input_Two : Inport  Port=2
  First wiper : Subsystem
  Secod wiper : Subsystem
  Wiper_Output_One : Outport
  Wiper_Output_Two : Outport  Port=2
  wires:
  Wiper_Input_One/1 -> First wiper/1(Input_one)
  First wiper/1(Output) -> Wiper_Output_One/1
  Secod wiper/1(Out1) -> Wiper_Output_Two/1
  Wiper_Input_Two/1 -> Secod wiper/1(Input_one)

== system Team6_1/BCM CAR/mirror ==
  note: Test Plan
  note: Sl No.
      | Test Cases
      | Input
      | output
      | Result
      |
      | 1.
      | tilt up
      | 1
      | tilt up
      | PASS
      |
      | 2.
      | tilt down
      | -1
      | tilt down
      | PASS
      |
      | 3.
      | pan right
      | 2
      | pan right
      | PASS
      |
      | 4.
      | pan down
      | -2
      | pan down
      | PASS
  note: Requirements:
      | Input:
      | Choose 1/-1 for tilt up/down
      | Choose 2/-2 for pan right/left
      | Output:
      | 1  ->  tilt up
      | 2  -> pan right
      | -1 -> tilt down
      | -2 -> pan down
  Input1 : Inport
  Input2 : Inport  Port=2
  Input3 : Inport  Port=3
  Input4 : Inport  Port=4
  left_mirror : Subsystem  TreatAsAtomicUnit=on
  right_mirror : Subsystem  TreatAsAtomicUnit=on
  Output28 : Outport
  Output29 : Outport  Port=2
  Output30 : Outport  Port=3
  Output31 : Outport  Port=4
  Output1 : Outport  Port=5
  Output2 : Outport  Port=6
  Output3 : Outport  Port=7
  Output4 : Outport  Port=8
  wires:
  Input2/1 -> right_mirror/1(Input2)
  right_mirror/2(Out2) -> Output29/1  "tilt_down"
  Input1/1 -> right_mirror/Enable
  right_mirror/4(Out4) -> Output31/1  "Pan_left"
  right_mirror/3(Output30) -> Output30/1  "Pan_Right"
  right_mirror/1(Tilt_up) -> Output28/1  "Tilt_up"
  left_mirror/2(Out2) -> Output2/1  "tilt_down"
  Input4/1 -> left_mirror/1(Input2)
  left_mirror/4(Out4) -> Output4/1  "Pan_left"
  left_mirror/1(Tilt_up) -> Output1/1  "Tilt_up"
  Input3/1 -> left_mirror/Enable
  left_mirror/3(Output30) -> Output3/1  "Pan_Right"

== system Team6_1/BCM CAR/power_window ==
  note: Requirements
      | There are 5 input signals for power_window subsystem
      | If lock input is enabled all the other signals won't work
      | Driver input has highest Priority over other passengers
      | All users can perform 4 actions: long press up, up, down, long press down
      | Expected output
      | Respective actions should be performed for all the user input
  Driver_input : Inport
  Passenger1_input : Inport  Port=2
  Passenger2_input : Inport  Port=3
  Passenger3_input : Inport  Port=4
  Enable : EnablePort
  Back_left_passenger : Subsystem
  Back_right_passenger : Subsystem
  Driver_priority : Logic  Operator=NOT  IconShape=distinctive  AllPortsSameDT=off  OutDataTypeStr=boolean
  driver_button : Subsystem
  front_passenger : Subsystem
  Out1 : Outport
  Out2 : Outport  Port=2
  Out3 : Outport  Port=3
  Out4 : Outport  Port=4
  wires:
  Driver_input/1 -> Driver_priority/1, driver_button/1(In1)  "Driver_input"
  driver_button/1(Out1) -> Out1/1  "Driver_output"
  front_passenger/1(Out1) -> Out2/1  "Passenger1_output"
  Back_right_passenger/1(Out1) -> Out4/1  "Passenger3_input"
  Back_left_passenger/1(Out1) -> Out3/1  "Passenger2_input"
  Driver_priority/1 -> Back_right_passenger/Enable, Back_left_passenger/Enable, front_passenger/Enable
  Passenger1_input/1 -> front_passenger/1(Input)
  Passenger3_input/1 -> Back_right_passenger/1(Input)
  Passenger2_input/1 -> Back_left_passenger/1(Input)

== system Team6_1/BCM CAR/External Light/Brake_subsystem ==
  In1 : Inport
  Logical Operator : Logic  AllPortsSameDT=off  OutDataTypeStr=boolean
  Signal Builder : Subsystem  Tag=STV Subsys  LoadFcn=sigbuilder_block('load');  StartFcn=sigbuilder_block('start');  StopFcn=sigbuilder_block('stop');  ClipboardFcn=sigbuilder_block('clipboard');  mask(Sigbuilder block){tuvar=[0:10]}
      mask help: Simulink:masks:SigbuilderBlock_MD
      mask init:
      | if ~strcmp(get_param(bdroot(gcbh),'SimulationStatus'),'stopped') tuvar = sigbuilder_block('maskInit'); end
      settings: CopyFcn=sigbuilder_block('copy');  DeleteFcn=sigbuilder_block('delete');  ModelCloseFcn=sigbuilder_block('modelClose');  PreSaveFcn=sigbuilder_block('preSave');  PauseFcn=sigbuilder_block('pause');  ContinueFcn=sigbuilder_block('continue');  NameChangeFcn=sigbuilder_block('namechange');  OpenFcn=sigbuilder_block('open',[437.6 153 550.4 359.25 ]);  CloseFcn=sigbuilder_block('close');
      mask Display: plot(0, 0, 100, 100,[2, 2, 32, 32, 2], [68, 8, 8, 68, 68],[32, 2], [38, 38], [32, 19, 2],[53, 60, 44], [32, 17, 17, 2],[16, 16, 31, 31]);txt = getActiveGroup(gcbh);text(2, 100, txt,'verticalAlignment', 'top');
  Out1 : Outport
  wires:
  Logical Operator/1 -> Out1/1
  Signal Builder/1(Signal 1) -> Logical Operator/1
  In1/1 -> Logical Operator/2

== system Team6_1/BCM CAR/External Light/Hazard_subsystem ==
  In1 : Inport
  AND : Logic  IconShape=distinctive  AllPortsSameDT=off  OutDataTypeStr=boolean
  Continuous Pulse Generator : DiscretePulseGenerator  PulseType=Time based  Period=1  PulseWidth=50
  Scope : Scope  NumInputPorts=2
  Triggered Subsystem : Subsystem  TreatAsAtomicUnit=on
  Out1 : Outport
  Out2 : Outport  Port=2
  Out3 : Outport  Port=3
  Out4 : Outport  Port=4
  wires:
  Triggered Subsystem/1(Out1) -> Out4/1, Out3/1, Out2/1, Scope/2, Out1/1
  Continuous Pulse Generator/1 -> AND/1, Triggered Subsystem/Trigger, Scope/1
  In1/1 -> AND/2
  AND/1 -> Triggered Subsystem/1(In1)

== system Team6_1/BCM CAR/External Light/If Action Subsystem ==
  In1 : Inport
  Action Port : ActionPort
  Out1 : Outport
  wires:
  In1/1 -> Out1/1

== system Team6_1/BCM CAR/External Light/Left_Indicator1 ==
  In1 : Inport
  AND : Logic  IconShape=distinctive  AllPortsSameDT=off  OutDataTypeStr=boolean
  Constant : Constant
  Out1 : Outport
  Out2 : Outport  Port=2
  wires:
  In1/1 -> AND/1
  Constant/1 -> AND/2
  AND/1 -> Out2/1, Out1/1

== system Team6_1/BCM CAR/External Light/Right_Indicator1 ==
  In1 : Inport
  AND : Logic  IconShape=distinctive  AllPortsSameDT=off  OutDataTypeStr=boolean
  Constant : Constant
  Out1 : Outport
  Out2 : Outport  Port=2
  wires:
  In1/1 -> AND/1
  Constant/1 -> AND/2
  AND/1 -> Out2/1, Out1/1

== system Team6_1/BCM CAR/External Light/front_light_left ==
  In1 : Inport
  Constant : Constant  Value=2
  Constant1 : Constant  Value=3
  Constant2 : Constant  Value=5
  Constant3 : Constant  Value=7
  High : RelationalOperator  Operator=<=  OutDataTypeStr=boolean  RndMeth=Simplest
  Low : RelationalOperator  Operator=>  OutDataTypeStr=boolean  RndMeth=Simplest
  Medium : Logic  IconShape=distinctive  AllPortsSameDT=off  OutDataTypeStr=boolean
  Relational Operator : RelationalOperator  Operator=<  OutDataTypeStr=boolean  RndMeth=Simplest
  Relational Operator3 : RelationalOperator  Operator=<=  OutDataTypeStr=boolean  RndMeth=Simplest
  Out1 : Outport
  Out2 : Outport  Port=2
  Out3 : Outport  Port=3
  wires:
  Constant/1 -> Low/1
  In1/1 -> High/2, Low/2, Relational Operator3/1, Relational Operator/2
  Low/1 -> Out1/1
  Constant1/1 -> Relational Operator/1
  Constant3/1 -> High/1
  High/1 -> Out3/1
  Relational Operator/1 -> Medium/1
  Relational Operator3/1 -> Medium/2
  Constant2/1 -> Relational Operator3/2
  Medium/1 -> Out2/1

== system Team6_1/BCM CAR/External Light/front_light_right ==
  In1 : Inport
  Constant : Constant  Value=2
  Constant1 : Constant  Value=3
  Constant2 : Constant  Value=5
  Constant3 : Constant  Value=7
  High : RelationalOperator  Operator=<=  OutDataTypeStr=boolean  RndMeth=Simplest
  Low : RelationalOperator  Operator=>  OutDataTypeStr=boolean  RndMeth=Simplest
  Medium : Logic  IconShape=distinctive  AllPortsSameDT=off  OutDataTypeStr=boolean
  Relational Operator : RelationalOperator  Operator=<  OutDataTypeStr=boolean  RndMeth=Simplest
  Relational Operator3 : RelationalOperator  Operator=<=  OutDataTypeStr=boolean  RndMeth=Simplest
  Out1 : Outport
  Out2 : Outport  Port=2
  Out3 : Outport  Port=3
  wires:
  Constant/1 -> Low/1
  In1/1 -> High/2, Low/2, Relational Operator3/1, Relational Operator/2
  Low/1 -> Out1/1
  Constant1/1 -> Relational Operator/1
  Constant3/1 -> High/1
  High/1 -> Out3/1
  Relational Operator/1 -> Medium/1
  Relational Operator3/1 -> Medium/2
  Constant2/1 -> Relational Operator3/2
  Medium/1 -> Out2/1

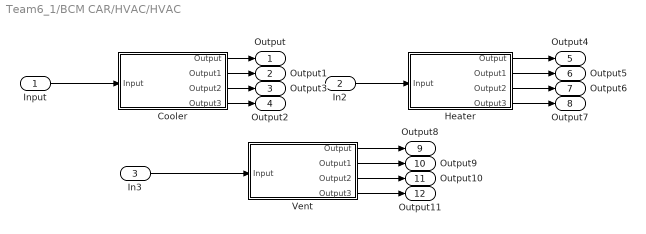
== system Team6_1/BCM CAR/HVAC/HVAC ==
  Input : Inport
  In2 : Inport  Port=2
  In3 : Inport  Port=3
  Cooler : Subsystem
  Heater : Subsystem
  Vent : Subsystem
  Output : Outport
  Output1 : Outport  Port=2
  Output3 : Outport  Port=3
  Output2 : Outport  Port=4
  Output4 : Outport  Port=5
  Output5 : Outport  Port=6
  Output6 : Outport  Port=7
  Output7 : Outport  Port=8
  Output8 : Outport  Port=9
  Output9 : Outport  Port=10
  Output10 : Outport  Port=11
  Output11 : Outport  Port=12
  wires:
  Input/1 -> Cooler/1(Input)
  In2/1 -> Heater/1(Input)
  In3/1 -> Vent/1(Input)
  Cooler/1(Output) -> Output/1
  Cooler/2(Output1) -> Output1/1
  Cooler/4(Output3) -> Output2/1
  Cooler/3(Output2) -> Output3/1
  Heater/1(Output) -> Output4/1
  Heater/2(Output1) -> Output5/1
  Heater/3(Output2) -> Output6/1
  Heater/4(Output3) -> Output7/1
  Vent/1(Output) -> Output8/1
  Vent/2(Output1) -> Output9/1
  Vent/3(Output2) -> Output10/1
  Vent/4(Output3) -> Output11/1

== system Team6_1/BCM CAR/Seat_subsystem/Front_Left ==
  note: Vertical Direction
  note: Horizontal Direction
  note: Test Case no
      | Input
      | Condition
      | Result
      |
      | 1
      | 0
      | Stay in current position
      | Pass
      |
      | 2
      | 1
      | Move in forward direction
      | Pass
      |
      | 3
      | -1
      | Move in backward Direction
      | Pass
  note: Test Plan
  note: Seat Subsystem Front Left
  note: Requirements:
      |
      | * The default position is selected if the user_input is 0.
      |
      | * For user input '1' the Seat moves Up in lean direction
      | and forward in height direction.
      |
      | For user input '-1' the Seat moves Downp in lean direction
      | and backward in height direction.
  note: Test Case no
      | Input
      | Condition
      | Result
      |
      | 4
      | 0
      | Stay in current position
      | Pass
      |
      | 5
      | 1
      | Move in forward direction
      | Pass
      |
      | 6
      | -1
      | Move in backward Direction
      | Pass
  Seat_i/p : Inport
  Horizontal_Direction : Subsystem  TreatAsAtomicUnit=on
  Vertical_Direction : Subsystem  TreatAsAtomicUnit=on
  mov_forw : Outport
  mov_back : Outport  Port=2
  stay_hor : Outport  Port=3
  mov_up : Outport  Port=4
  mov_down : Outport  Port=5
  stay_ver : Outport  Port=6
  wires:
  Vertical_Direction/1(mov_up) -> mov_up/1  "move_up"
  Vertical_Direction/2(mov_down) -> mov_down/1  "move_down"
  Horizontal_Direction/2(mov_back) -> mov_back/1  "move_backward"
  Vertical_Direction/3(stay) -> stay_ver/1  "current_position"
  Seat_i/p/1 -> Horizontal_Direction/1(In1), Vertical_Direction/1(user_input)  "User_input"
  Horizontal_Direction/1(mov_for) -> mov_forw/1  "move_forward"
  Horizontal_Direction/3(stay) -> stay_hor/1  "current_position"

== system Team6_1/BCM CAR/Seat_subsystem/Front_Right ==
  note: Seat Subsystem Front Right
  note: Requirements:
      |
      | * The default position is selected if the user_input is 0.
      |
      | * For user input '1' the Seat moves Up in lean direction
      | and forward in height direction.
      |
      | For user input '-1' the Seat moves Downp in lean direction
      | and backward in height direction.
  note: Test Case no
      | Input
      | Condition
      | Result
      |
      | 1
      | 0
      | Stay in current position
      | Pass
      |
      | 2
      | 1
      | Move in forward direction
      | Pass
      |
      | 3
      | -1
      | Move in backward Direction
      | Pass
  note: Test Plan
  note: Test Case no
      | Input
      | Condition
      | Result
      |
      | 4
      | 0
      | Stay in current position
      | Pass
      |
      | 5
      | 1
      | Move in forward direction
      | Pass
      |
      | 6
      | -1
      | Move in backward Direction
      | Pass
  note: Horizontal Direction
  note: Vertical Direction
  Seat_i/p : Inport
  Horizontal_Direction : Subsystem  TreatAsAtomicUnit=on
  Vertical_Direction : Subsystem  TreatAsAtomicUnit=on
  mov_forw : Outport
  mov_back : Outport  Port=2
  stay_hor : Outport  Port=3
  mov_up : Outport  Port=4
  mov_down : Outport  Port=5
  stay_ver : Outport  Port=6
  wires:
  Vertical_Direction/1(mov_up) -> mov_up/1  "move_up"
  Vertical_Direction/2(mov_back) -> mov_down/1  "move_down"
  Vertical_Direction/3(stay) -> stay_ver/1  "current_position"
  Seat_i/p/1 -> Horizontal_Direction/1(In1), Vertical_Direction/1(user_input)  "User_input"
  Horizontal_Direction/1(mov_for) -> mov_forw/1  "move_forward"
  Horizontal_Direction/2(mov_back) -> mov_back/1  "move_backward"
  Horizontal_Direction/3(stay) -> stay_hor/1  "current_position"

== system Team6_1/BCM CAR/Wiper Subsystem/First wiper ==
  Input_one : Inport
  If Action Subsystem : Subsystem  TreatAsAtomicUnit=on
  If Action Subsystem1 : Subsystem  TreatAsAtomicUnit=on
  If Action Subsystem2 : Subsystem  TreatAsAtomicUnit=on
  If Action Subsystem3 : Subsystem  TreatAsAtomicUnit=on
  Input Gain : Gain  Gain=20
  Signal Generator : SignalGenerator  Units=rad/sec
  Signal Generator1 : SignalGenerator  Frequency=2  Units=rad/sec
  Signal Generator2 : SignalGenerator  Frequency=3  Units=rad/sec
  Signal Generator3 : SignalGenerator  Units=rad/sec
  if else block : If  IfExpression=u1<=20  ElseIfExpressions=u1<=40,u1<=60
  "merging the data " : Merge  Inputs=4
  Output : Outport
  wires:
  if else block/2 -> If Action Subsystem1/Action  "if input == 40"
  If Action Subsystem3/1(Out1) -> "merging the data "/4
  if else block/1 -> If Action Subsystem/Action  "If input == 20"
  if else block/3 -> If Action Subsystem2/Action  "if input == 60"
  Signal Generator2/1 -> If Action Subsystem3/1(In1)
  If Action Subsystem/1(Out1) -> "merging the data "/1
  Signal Generator1/1 -> If Action Subsystem2/1(In1)
  If Action Subsystem1/1(Out1) -> "merging the data "/2
  Input Gain/1 -> if else block/1
  If Action Subsystem2/1(Out1) -> "merging the data "/3
  "merging the data "/1 -> Output/1
  Input_one/1 -> Input Gain/1
  Signal Generator/1 -> If Action Subsystem1/1(In1)
  Signal Generator3/1 -> If Action Subsystem/1(In1)
  if else block/4 -> If Action Subsystem3/Action  "if input ==0"

== system Team6_1/BCM CAR/Wiper Subsystem/Secod wiper ==
  Input_one : Inport
  If Action Subsystem : Subsystem  TreatAsAtomicUnit=on
  If Action Subsystem1 : Subsystem  TreatAsAtomicUnit=on
  If Action Subsystem2 : Subsystem  TreatAsAtomicUnit=on
  If Action Subsystem3 : Subsystem  TreatAsAtomicUnit=on
  Input Gain : Gain  Gain=20
  Signal Generator : SignalGenerator  Units=rad/sec
  Signal Generator1 : SignalGenerator  Frequency=2  Units=rad/sec
  Signal Generator2 : SignalGenerator  Frequency=3  Units=rad/sec
  Signal Generator3 : SignalGenerator  Units=rad/sec
  if else block : If  IfExpression=u1<=20  ElseIfExpressions=u1<=40,u1<=60
  "merging the data " : Merge  Inputs=4
  Out1 : Outport
  wires:
  if else block/2 -> If Action Subsystem1/Action  "if input == 40"
  If Action Subsystem3/1(Out1) -> "merging the data "/4
  if else block/1 -> If Action Subsystem/Action  "If input == 20"
  if else block/3 -> If Action Subsystem2/Action  "if input == 60"
  Signal Generator2/1 -> If Action Subsystem3/1(In1)
  If Action Subsystem/1(Out1) -> "merging the data "/1
  Signal Generator1/1 -> If Action Subsystem2/1(In1)
  If Action Subsystem1/1(Out1) -> "merging the data "/2
  Input Gain/1 -> if else block/1
  If Action Subsystem2/1(Out1) -> "merging the data "/3
  "merging the data "/1 -> Out1/1
  Input_one/1 -> Input Gain/1
  Signal Generator/1 -> If Action Subsystem1/1(In1)
  Signal Generator3/1 -> If Action Subsystem/1(In1)
  if else block/4 -> If Action Subsystem3/Action  "if input ==0"

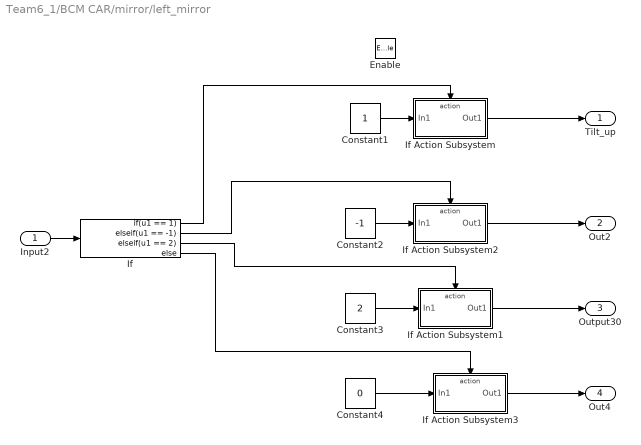
== system Team6_1/BCM CAR/mirror/left_mirror ==
  Input2 : Inport
  Enable : EnablePort
  Constant1 : Constant
  Constant2 : Constant  Value=-1
  Constant3 : Constant  Value=2
  Constant4 : Constant  Value=0
  If : If  IfExpression=u1 == 1  ElseIfExpressions=u1 == -1 , u1 == 2
  If Action Subsystem : Subsystem  TreatAsAtomicUnit=on
  If Action Subsystem1 : Subsystem  TreatAsAtomicUnit=on
  If Action Subsystem2 : Subsystem  TreatAsAtomicUnit=on
  If Action Subsystem3 : Subsystem  TreatAsAtomicUnit=on
  Tilt_up : Outport
  Out2 : Outport  Port=2
  Output30 : Outport  Port=3
  Out4 : Outport  Port=4
  wires:
  If/1 -> If Action Subsystem/Action
  If/2 -> If Action Subsystem2/Action
  If/3 -> If Action Subsystem1/Action
  If/4 -> If Action Subsystem3/Action
  Constant1/1 -> If Action Subsystem/1(In1)
  If Action Subsystem/1(Out1) -> Tilt_up/1
  Constant2/1 -> If Action Subsystem2/1(In1)
  Constant3/1 -> If Action Subsystem1/1(In1)
  Constant4/1 -> If Action Subsystem3/1(In1)
  If Action Subsystem2/1(Out1) -> Out2/1
  If Action Subsystem1/1(Out1) -> Output30/1
  If Action Subsystem3/1(Out1) -> Out4/1
  Input2/1 -> If/1

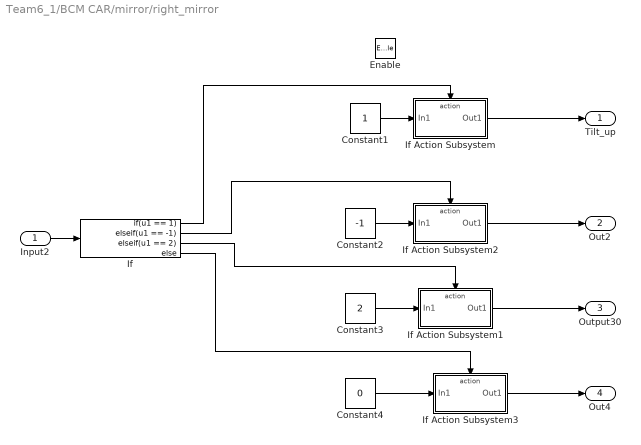
== system Team6_1/BCM CAR/mirror/right_mirror ==
  Input2 : Inport
  Enable : EnablePort
  Constant1 : Constant
  Constant2 : Constant  Value=-1
  Constant3 : Constant  Value=2
  Constant4 : Constant  Value=0
  If : If  IfExpression=u1 == 1  ElseIfExpressions=u1 == -1 , u1 == 2
  If Action Subsystem : Subsystem  TreatAsAtomicUnit=on
  If Action Subsystem1 : Subsystem  TreatAsAtomicUnit=on
  If Action Subsystem2 : Subsystem  TreatAsAtomicUnit=on
  If Action Subsystem3 : Subsystem  TreatAsAtomicUnit=on
  Tilt_up : Outport
  Out2 : Outport  Port=2
  Output30 : Outport  Port=3
  Out4 : Outport  Port=4
  wires:
  If/1 -> If Action Subsystem/Action
  If/2 -> If Action Subsystem2/Action
  If/3 -> If Action Subsystem1/Action
  If/4 -> If Action Subsystem3/Action
  Constant1/1 -> If Action Subsystem/1(In1)
  If Action Subsystem/1(Out1) -> Tilt_up/1
  Constant2/1 -> If Action Subsystem2/1(In1)
  Constant3/1 -> If Action Subsystem1/1(In1)
  Constant4/1 -> If Action Subsystem3/1(In1)
  If Action Subsystem2/1(Out1) -> Out2/1
  If Action Subsystem1/1(Out1) -> Output30/1
  If Action Subsystem3/1(Out1) -> Out4/1
  Input2/1 -> If/1

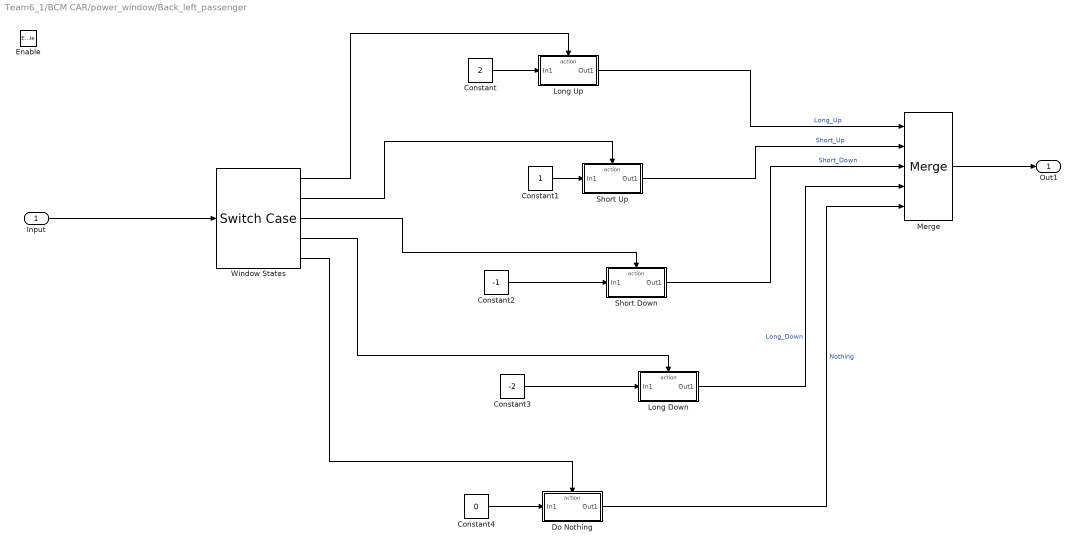
== system Team6_1/BCM CAR/power_window/Back_left_passenger ==
  Input : Inport
  Enable : EnablePort
  Constant : Constant  Value=2
  Constant1 : Constant
  Constant2 : Constant  Value=-1
  Constant3 : Constant  Value=-2
  Constant4 : Constant  Value=0
  Do Nothing : Subsystem  TreatAsAtomicUnit=on
  Long Down : Subsystem  TreatAsAtomicUnit=on
  Long Up : Subsystem  TreatAsAtomicUnit=on
  Merge : Merge  Inputs=5
  Short Down : Subsystem  TreatAsAtomicUnit=on
  Short Up : Subsystem  TreatAsAtomicUnit=on
  Window States : SwitchCase  CaseConditions={1,2,3,4}
  Out1 : Outport
  wires:
  Long Up/1(Out1) -> Merge/1  "Long_Up"
  Window States/5 -> Do Nothing/Action
  Input/1 -> Window States/1
  Short Down/1(Out1) -> Merge/3  "Short_Down"
  Window States/3 -> Short Down/Action
  Constant1/1 -> Short Up/1(In1)
  Merge/1 -> Out1/1
  Window States/1 -> Long Up/Action
  Window States/2 -> Short Up/Action
  Do Nothing/1(Out1) -> Merge/5  "Nothing"
  Short Up/1(Out1) -> Merge/2  "Short_Up"
  Long Down/1(Out1) -> Merge/4  "Long_Down"
  Constant4/1 -> Do Nothing/1(In1)
  Window States/4 -> Long Down/Action
  Constant/1 -> Long Up/1(In1)
  Constant3/1 -> Long Down/1(In1)
  Constant2/1 -> Short Down/1(In1)

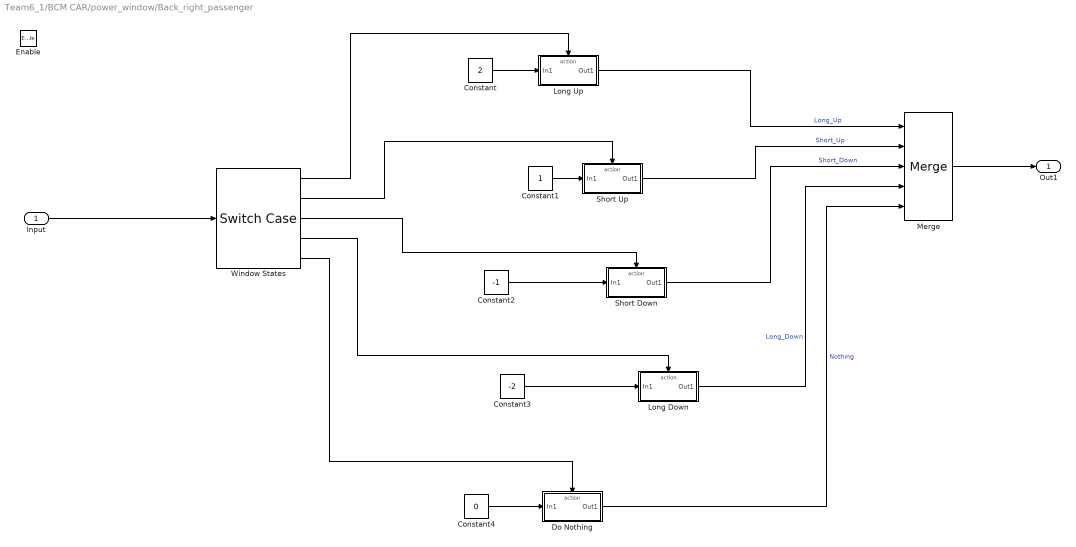
== system Team6_1/BCM CAR/power_window/Back_right_passenger ==
  Input : Inport
  Enable : EnablePort
  Constant : Constant  Value=2
  Constant1 : Constant
  Constant2 : Constant  Value=-1
  Constant3 : Constant  Value=-2
  Constant4 : Constant  Value=0
  Do Nothing : Subsystem  TreatAsAtomicUnit=on
  Long Down : Subsystem  TreatAsAtomicUnit=on
  Long Up : Subsystem  TreatAsAtomicUnit=on
  Merge : Merge  Inputs=5
  Short Down : Subsystem  TreatAsAtomicUnit=on
  Short Up : Subsystem  TreatAsAtomicUnit=on
  Window States : SwitchCase  CaseConditions={1,2,3,4}
  Out1 : Outport
  wires:
  Long Up/1(Out1) -> Merge/1  "Long_Up"
  Window States/5 -> Do Nothing/Action
  Input/1 -> Window States/1
  Short Down/1(Out1) -> Merge/3  "Short_Down"
  Window States/3 -> Short Down/Action
  Constant1/1 -> Short Up/1(In1)
  Merge/1 -> Out1/1
  Window States/1 -> Long Up/Action
  Window States/2 -> Short Up/Action
  Do Nothing/1(Out1) -> Merge/5  "Nothing"
  Short Up/1(Out1) -> Merge/2  "Short_Up"
  Long Down/1(Out1) -> Merge/4  "Long_Down"
  Constant4/1 -> Do Nothing/1(In1)
  Window States/4 -> Long Down/Action
  Constant/1 -> Long Up/1(In1)
  Constant3/1 -> Long Down/1(In1)
  Constant2/1 -> Short Down/1(In1)

== system Team6_1/BCM CAR/power_window/driver_button ==
  In1 : Inport
  Do_Nothing : Subsystem  TreatAsAtomicUnit=on
  Long_Down : Subsystem  TreatAsAtomicUnit=on
  Long_Down_ip : Constant  Value=-2
  Long_Up : Subsystem  TreatAsAtomicUnit=on
  Long_Up_ip : Constant  Value=2
  Merge : Merge  Inputs=5
  Short_Down : Subsystem  TreatAsAtomicUnit=on
  Short_Down_ip : Constant  Value=-1
  Short_Up : Subsystem  TreatAsAtomicUnit=on
  Short_Up_ip : Constant
  Window States : SwitchCase  CaseConditions={1,2,3,4}
  default : Constant  Value=0
  Out1 : Outport
  wires:
  Long_Up/1(Out1) -> Merge/1  "Long_Up_op"
  Window States/5 -> Do_Nothing/Action
  In1/1 -> Window States/1
  Short_Down/1(Out1) -> Merge/3  "Short_Down_op"
  Window States/3 -> Short_Down/Action
  Short_Up_ip/1 -> Short_Up/1(In1)
  Merge/1 -> Out1/1
  Window States/1 -> Long_Up/Action
  Window States/2 -> Short_Up/Action
  Do_Nothing/1(Out1) -> Merge/5  "Nothing"
  Short_Up/1(Out1) -> Merge/2  "Short_Up_op"
  Long_Down/1(Out1) -> Merge/4  "Long_Down_op"
  default/1 -> Do_Nothing/1(In1)
  Window States/4 -> Long_Down/Action
  Long_Up_ip/1 -> Long_Up/1(In1)
  Long_Down_ip/1 -> Long_Down/1(In1)
  Short_Down_ip/1 -> Short_Down/1(In1)

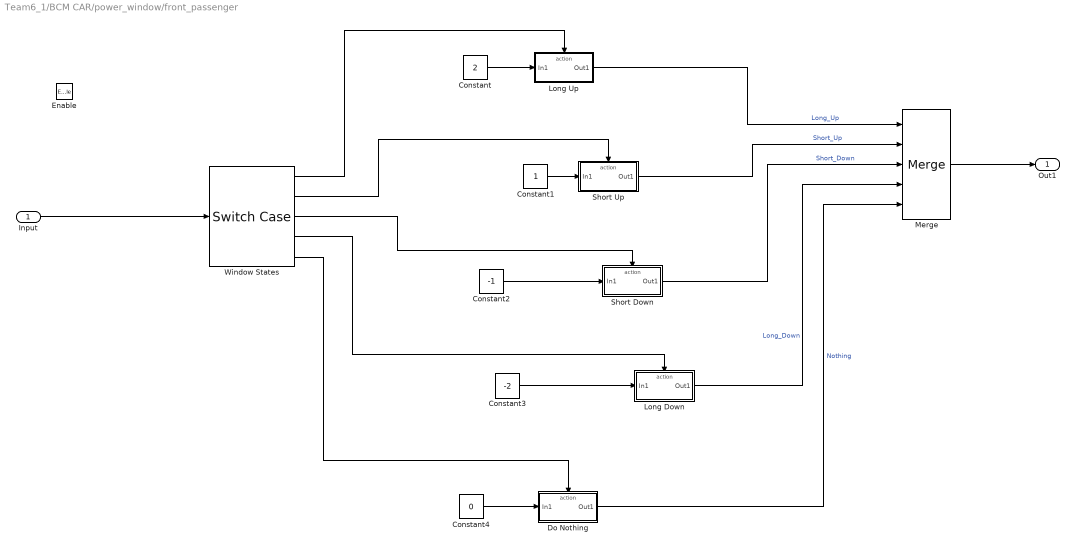
== system Team6_1/BCM CAR/power_window/front_passenger ==
  Input : Inport
  Enable : EnablePort
  Constant : Constant  Value=2
  Constant1 : Constant
  Constant2 : Constant  Value=-1
  Constant3 : Constant  Value=-2
  Constant4 : Constant  Value=0
  Do Nothing : Subsystem  TreatAsAtomicUnit=on
  Long Down : Subsystem  TreatAsAtomicUnit=on
  Long Up : Subsystem  TreatAsAtomicUnit=on
  Merge : Merge  Inputs=5
  Short Down : Subsystem  TreatAsAtomicUnit=on
  Short Up : Subsystem  TreatAsAtomicUnit=on
  Window States : SwitchCase  CaseConditions={1,2,3,4}
  Out1 : Outport
  wires:
  Long Up/1(Out1) -> Merge/1  "Long_Up"
  Window States/5 -> Do Nothing/Action
  Input/1 -> Window States/1
  Short Down/1(Out1) -> Merge/3  "Short_Down"
  Window States/3 -> Short Down/Action
  Constant1/1 -> Short Up/1(In1)
  Merge/1 -> Out1/1
  Window States/1 -> Long Up/Action
  Window States/2 -> Short Up/Action
  Do Nothing/1(Out1) -> Merge/5  "Nothing"
  Short Up/1(Out1) -> Merge/2  "Short_Up"
  Long Down/1(Out1) -> Merge/4  "Long_Down"
  Constant4/1 -> Do Nothing/1(In1)
  Window States/4 -> Long Down/Action
  Constant/1 -> Long Up/1(In1)
  Constant3/1 -> Long Down/1(In1)
  Constant2/1 -> Short Down/1(In1)

== system Team6_1/BCM CAR/External Light/Brake_subsystem/Signal Builder ==
  Demux : Demux  Tag=STV Demux  Outputs=1
      settings: DisplayOption=none
  FromWs : FromWorkspace  Tag=STV FromWs  VariableName=tuvar
      SigBuilderData=|
      | common.afterFinalStr = 'Extrapolate'
      | common.sampleTime = 0
      | dataSet.timeRange = [0 10]
      | dataSet.name = 'Group 1'
      | sbobj.Groups.Name = 'Group 1'
      | sbobj.Groups.Signals.Name = 'Signal 1'
      | sbobj.Groups.Signals.XData = [0 3 3 6 6 10]
      | sbobj.Groups.Signals.YData = [0 0 1 1 0 0]
  Signal 1 : Outport  Tag=STV Outport
  wires:
  Demux/1 -> Signal 1/1
  FromWs/1 -> Demux/1

== system Team6_1/BCM CAR/External Light/Hazard_subsystem/Triggered Subsystem ==
  In1 : Inport
  Trigger : TriggerPort  TriggerType=either  VariantControl=Variant
  Out1 : Outport
  wires:
  In1/1 -> Out1/1

== system Team6_1/BCM CAR/HVAC/HVAC/Cooler ==
  Input : Inport
  Constant : Constant
  Constant1 : Constant  Value=0
  Constant2 : Constant
  Constant3 : Constant
  If : If  IfExpression=u1 == 1  ElseIfExpressions=u1 == 2, u1 == 3
  If Action Subsystem : Subsystem  TreatAsAtomicUnit=on
  If Action Subsystem1 : Subsystem  TreatAsAtomicUnit=on
  If Action Subsystem2 : Subsystem  TreatAsAtomicUnit=on
  If Action Subsystem3 : Subsystem  TreatAsAtomicUnit=on
  Output : Outport
  Output1 : Outport  Port=2
  Output2 : Outport  Port=3
  Output3 : Outport  Port=4
  wires:
  If/4 -> If Action Subsystem3/Action
  If/1 -> If Action Subsystem/Action
  If/3 -> If Action Subsystem2/Action
  If Action Subsystem3/1(Out1) -> Output3/1
  If Action Subsystem1/1(Output1) -> Output1/1
  Constant1/1 -> If Action Subsystem3/1(In1)
  If Action Subsystem2/1(Out1) -> Output2/1
  If Action Subsystem/1(Out1) -> Output/1  "if input = 1"
  Input/1 -> If/1
  If/2 -> If Action Subsystem1/Action
  Constant/1 -> If Action Subsystem/1(In1)
  Constant2/1 -> If Action Subsystem1/1(In1)
  Constant3/1 -> If Action Subsystem2/1(In1)

== system Team6_1/BCM CAR/HVAC/HVAC/Heater ==
  Input : Inport
  Constant : Constant
  Constant1 : Constant  Value=0
  If : If  IfExpression=u1 == 1  ElseIfExpressions=u1 == 2, u1 == 3
  If Action Subsystem : Subsystem  TreatAsAtomicUnit=on
  If Action Subsystem1 : Subsystem  TreatAsAtomicUnit=on
  If Action Subsystem2 : Subsystem  TreatAsAtomicUnit=on
  If Action Subsystem3 : Subsystem  TreatAsAtomicUnit=on
  Signal Builder1 : Subsystem  Tag=STV Subsys  LoadFcn=sigbuilder_block('load');  StartFcn=sigbuilder_block('start');  StopFcn=sigbuilder_block('stop');  ClipboardFcn=sigbuilder_block('clipboard');  mask(Sigbuilder block){tuvar=[0:10]}
      mask help: Simulink:masks:SigbuilderBlock_MD
      mask init:
      | if ~strcmp(get_param(bdroot(gcbh),'SimulationStatus'),'stopped') tuvar = sigbuilder_block('maskInit'); end
      settings: CopyFcn=sigbuilder_block('copy');  DeleteFcn=sigbuilder_block('delete');  ModelCloseFcn=sigbuilder_block('modelClose');  PreSaveFcn=sigbuilder_block('preSave');  PauseFcn=sigbuilder_block('pause');  ContinueFcn=sigbuilder_block('continue');  NameChangeFcn=sigbuilder_block('namechange');  OpenFcn=sigbuilder_block('open',[437.6 153 550.4 359.25 ]);  CloseFcn=sigbuilder_block('close');
      mask Display: plot(0, 0, 100, 100,[2, 2, 32, 32, 2], [68, 8, 8, 68, 68],[32, 2], [38, 38], [32, 19, 2],[53, 60, 44], [32, 17, 17, 2],[16, 16, 31, 31]);txt = getActiveGroup(gcbh);text(2, 100, txt,'verticalAlignment', 'top');
  Signal Builder2 : Subsystem  Tag=STV Subsys  LoadFcn=sigbuilder_block('load');  StartFcn=sigbuilder_block('start');  StopFcn=sigbuilder_block('stop');  ClipboardFcn=sigbuilder_block('clipboard');  mask(Sigbuilder block){tuvar=[0:10]}
      mask help: Simulink:masks:SigbuilderBlock_MD
      mask init:
      | if ~strcmp(get_param(bdroot(gcbh),'SimulationStatus'),'stopped') tuvar = sigbuilder_block('maskInit'); end
      settings: CopyFcn=sigbuilder_block('copy');  DeleteFcn=sigbuilder_block('delete');  ModelCloseFcn=sigbuilder_block('modelClose');  PreSaveFcn=sigbuilder_block('preSave');  PauseFcn=sigbuilder_block('pause');  ContinueFcn=sigbuilder_block('continue');  NameChangeFcn=sigbuilder_block('namechange');  OpenFcn=sigbuilder_block('open',[437.6 153 550.4 359.25 ]);  CloseFcn=sigbuilder_block('close');
      mask Display: plot(0, 0, 100, 100,[2, 2, 32, 32, 2], [68, 8, 8, 68, 68],[32, 2], [38, 38], [32, 19, 2],[53, 60, 44], [32, 17, 17, 2],[16, 16, 31, 31]);txt = getActiveGroup(gcbh);text(2, 100, txt,'verticalAlignment', 'top');
  Output : Outport
  Output1 : Outport  Port=2
  Output2 : Outport  Port=3
  Output3 : Outport  Port=4
  wires:
  If/4 -> If Action Subsystem3/Action
  If/2 -> If Action Subsystem1/Action
  Signal Builder2/1(Signal 1) -> If Action Subsystem2/1(In1)
  If Action Subsystem2/1(Out1) -> Output2/1
  Constant1/1 -> If Action Subsystem3/1(In1)
  If Action Subsystem3/1(Out1) -> Output3/1
  Input/1 -> If/1
  Constant/1 -> If Action Subsystem/1(In1)
  If/3 -> If Action Subsystem2/Action
  If/1 -> If Action Subsystem/Action
  If Action Subsystem1/1(Out1) -> Output1/1
  Signal Builder1/1(Signal 2) -> If Action Subsystem1/1(In1)
  If Action Subsystem/1(Output) -> Output/1
